simulink model "Cooperative_XeYe"  (Simulink 9.1)
settings: Solver=ode45  StartTime=0.0  StopTime=800  FixedStep=0.2  RelTol=1e-3
values from neighbouring files (symbols this model uses):
  A1 = 0.08    [Parameters.m]
  a1 = 10    [Parameters.m]
  A2 = 0.08    [Parameters.m]
  a2 = 10    [Parameters.m]
  A3 = 0.08    [Parameters.m]
  a3 = 10    [Parameters.m]
  H_A = 2.0    (= 2)    [Parameters.m]
  H_B = 2.0    (= 2)    [Parameters.m]
  k1_A = 5    [Parameters.m]
  k1_B = 0.1    [Parameters.m]
  k1_C = 5    [Parameters.m]
  k_update_A = 5.0    (= 5)    [Parameters.m]
  k_update_B = 10.0    (= 10)    [Parameters.m]
  k_update_C = 5.0    (= 5)    [Parameters.m]
  T = 0.2    [Parameters.m]
  v_0 = 1.0    (= 1)    [Parameters.m]
settings Model: Creator=sunky  LastModifiedBy=xiaobo
settings DataIOCC: SaveFormat=Dataset
settings OptimizationCC: LifeSpan=auto
settings DebuggingCC: UnderspecifiedInitializationDetection=Simplified  MergeDetectMultiDrivingBlocksExec=error  SFUnexpectedBacktrackingDiag=error  SFNoUnconditionalDefaultTransitionDiag=error  SFExecutionAtInitializationDiag=warning
settings HardwareCC: ProdBitPerPointer=64  ProdBitPerSizeT=64  ProdBitPerPtrDiffT=64  ProdLargestAtomicFloat=Float  ProdIntDivRoundTo=Zero  ProdEndianess=LittleEndian  ProdWordSize=64  ProdHWDeviceType=Intel->x86-64 (Windows64)
settings ModelReferenceCC: PropagateSignalLabelsOutOfModel=on
settings GRTTargetCC: TargetLangStandard=C99 (ISO)  CombineOutputUpdateFcns=on  GRTInterface=off
settings ConfigComp: CovMetricSettings=dwe  CovHtmlReporting=off  CovSaveCumulativeToWorkspaceVar=off  CovSaveSingleToWorkspaceVar=off  CovExternalEMLEnable=on

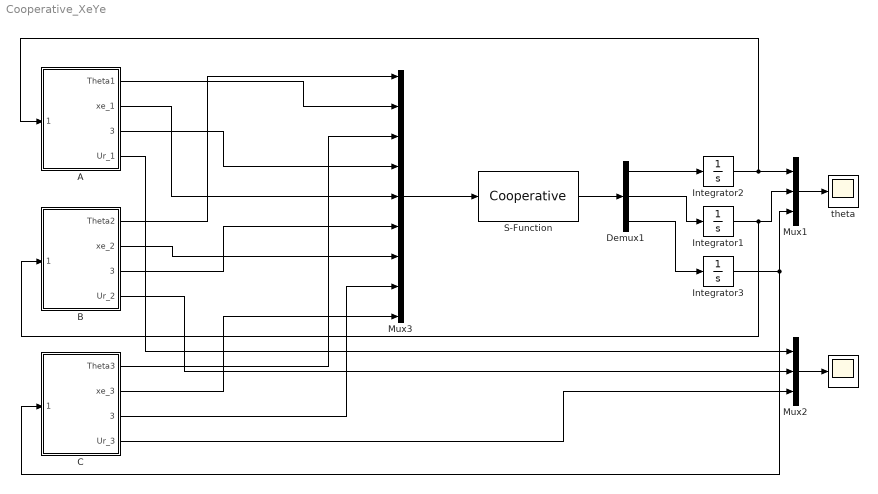
== system Cooperative_XeYe ==
  "   " : Scope
  " theta " : Scope
  A : Subsystem
  B : Subsystem
  C : Subsystem
  Demux1 : Demux  Outputs=3
  Integrator1 : Integrator
  Integrator2 : Integrator
  Integrator3 : Integrator
  Mux1 : Mux  Inputs=3
  Mux2 : Mux  Inputs=3
  Mux3 : Mux  Inputs=9
  S-Function : S-Function  FunctionName=Cooperative  Parameters=A1,A2,A3,v_0,T,a1,a2,a3  SFunctionDeploymentMode=off  EnableBusSupport=off
  wires:
  A/2(xe_1) -> Mux3/5
  A/3(u_dxing_A) -> Mux3/4
  B/2(xe_2) -> Mux3/7
  B/3(u_dxing_B) -> Mux3/6
  C/2(xe_3) -> Mux3/9
  C/3(u_dxing_C) -> Mux3/8
  Mux3/1 -> S-Function/1
  S-Function/1 -> Demux1/1
  Demux1/1 -> Integrator2/1
  Demux1/2 -> Integrator1/1
  Demux1/3 -> Integrator3/1
  Integrator2/1 -> A/1(Update1), Mux1/1
  Integrator1/1 -> B/1(Update2), Mux1/2
  Integrator3/1 -> C/1(Update3), Mux1/3
  Mux1/1 -> " theta "/1
  A/4(Ur_1) -> Mux2/1
  B/4(Ur_2) -> Mux2/2
  C/4(Ur_3) -> Mux2/3
  Mux2/1 -> "   "/1
  A/1(Theta1) -> Mux3/2
  B/1(Theta2) -> Mux3/1
  C/1(Theta3) -> Mux3/3

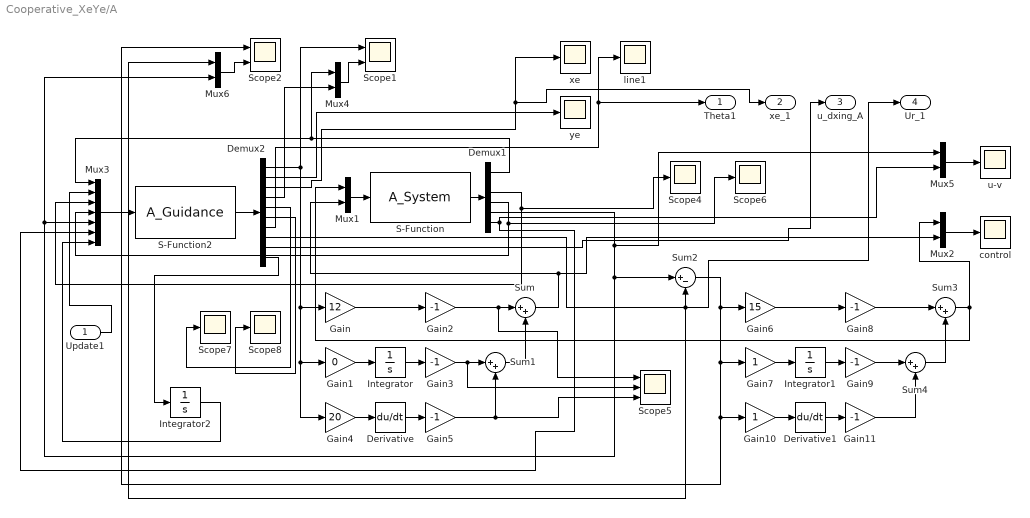
== system Cooperative_XeYe/A ==
  Update1 : Inport
  Demux1 : Demux  Outputs=6
  Demux2 : Demux  Outputs=10
  Derivative : Derivative
  Derivative1 : Derivative
  Gain : Gain  Gain=12
  Gain1 : Gain  Gain=0
  Gain10 : Gain
  Gain{2..3,5,8..9,11} (6 alike) : Gain  Gain=-1
  Gain4 : Gain  Gain=20
  Gain6 : Gain  Gain=15
  Gain7 : Gain
  Integrator : Integrator
  Integrator1 : Integrator
  Integrator2 : Integrator
  Mux{1..2,4..6} (5 alike) : Mux  Inputs=2
  Mux3 : Mux  Inputs=7
  S-Function : S-Function  FunctionName=A_System  SFunctionDeploymentMode=off  EnableBusSupport=off
  S-Function2 : S-Function  FunctionName=A_Guidance  Parameters=H_A,v_0,k_update_A,k1_A  SFunctionDeploymentMode=off  EnableBusSupport=off
  Scope1 : Scope  NumInputPorts=2
  Scope2 : Scope  NumInputPorts=2
  Scope{4,6..8} (4 alike) : Scope
  Scope5 : Scope  NumInputPorts=3
  Sum{,1,3..4} (4 alike) : Sum  Inputs=|++
  Sum2 : Sum  Inputs=|+-
  control : Scope
  line1 : Scope
  u-v : Scope
  xe : Scope
  ye : Scope
  Theta1 : Outport
  xe_1 : Outport  Port=2
  u_dxing_A : Outport  Port=3
  Ur_1 : Outport  Port=4
  wires:
  Demux1/1 -> Mux4/1, Mux3/1
  Gain8/1 -> Sum3/1
  Derivative1/1 -> Gain11/1
  Mux3/1 -> S-Function2/1
  S-Function/1 -> Demux1/1
  Demux2/5 -> Scope7/1
  Integrator1/1 -> Gain9/1
  Gain6/1 -> Gain8/1
  Gain5/1 -> Sum1/2, Scope5/3
  Sum/1 -> Mux2/2, Mux1/2
  Mux2/1 -> control/1
  Gain3/1 -> Scope5/2, Sum1/1
  Gain2/1 -> Scope5/1, Sum/1
  Demux2/6 -> Scope8/1
  Sum2/1 -> Scope2/1, Gain10/1, Gain7/1, Gain6/1
  Gain7/1 -> Integrator1/1
  Demux2/8 -> Ur_1/1, Mux6/1, Sum2/2
  Demux1/5 -> Mux5/1, Sum2/1, Mux6/2, Mux3/5
  Sum3/1 -> Mux1/1, Mux2/1
  Gain9/1 -> Sum4/1
  Mux1/1 -> S-Function/1
  Demux2/7 -> Theta1/1, line1/1
  Gain10/1 -> Derivative1/1
  Demux1/4 -> Scope6/1, Mux3/4
  S-Function2/1 -> Demux2/1
  Integrator/1 -> Gain3/1
  Demux1/6 -> Mux3/6, Mux5/2
  Gain/1 -> Gain2/1
  Gain11/1 -> Sum4/2
  Demux2/3 -> xe_1/1, xe/1
  Mux5/1 -> u-v/1
  Demux2/9 -> u_dxing_A/1
  Mux4/1 -> Scope1/2
  Gain4/1 -> Derivative/1
  Derivative/1 -> Gain5/1
  Gain1/1 -> Integrator/1
  Mux6/1 -> Scope2/2
  Demux2/4 -> Mux4/2
  Demux2/1 -> Scope1/1, Gain4/1, Gain1/1, Gain/1
  Sum1/1 -> Sum/2
  Demux2/2 -> ye/1
  Demux1/3 -> Scope4/1, Mux3/3
  Sum4/1 -> Sum3/2
  Demux2/10 -> Integrator2/1
  Integrator2/1 -> Mux3/7
  Update1/1 -> Mux3/2

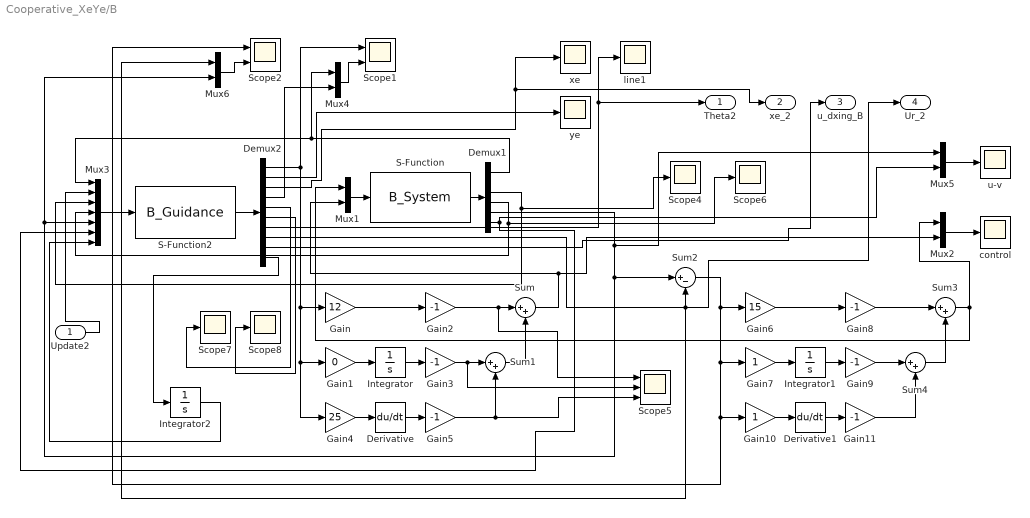
== system Cooperative_XeYe/B ==
  Update2 : Inport
  Demux1 : Demux  Outputs=6
  Demux2 : Demux  Outputs=10
  Derivative : Derivative
  Derivative1 : Derivative
  Gain : Gain  Gain=12
  Gain1 : Gain  Gain=0
  Gain10 : Gain
  Gain{2..3,5,8..9,11} (6 alike) : Gain  Gain=-1
  Gain4 : Gain  Gain=25
  Gain6 : Gain  Gain=15
  Gain7 : Gain
  Integrator : Integrator
  Integrator1 : Integrator
  Integrator2 : Integrator
  Mux{1..2,4..6} (5 alike) : Mux  Inputs=2
  Mux3 : Mux  Inputs=7
  S-Function : S-Function  FunctionName=B_System  SFunctionDeploymentMode=off  EnableBusSupport=off
  S-Function2 : S-Function  FunctionName=B_Guidance  Parameters=H_B,v_0,k_update_B,k1_B  SFunctionDeploymentMode=off  EnableBusSupport=off
  Scope1 : Scope  NumInputPorts=2
  Scope2 : Scope  NumInputPorts=2
  Scope{4,6..8} (4 alike) : Scope
  Scope5 : Scope  NumInputPorts=3
  Sum{,1,3..4} (4 alike) : Sum  Inputs=|++
  Sum2 : Sum  Inputs=|+-
  control : Scope
  line1 : Scope
  u-v : Scope
  xe : Scope
  ye : Scope
  Theta2 : Outport
  xe_2 : Outport  Port=2
  u_dxing_B : Outport  Port=3
  Ur_2 : Outport  Port=4
  wires:
  Demux1/1 -> Mux4/1, Mux3/1
  Gain8/1 -> Sum3/1
  Derivative1/1 -> Gain11/1
  Mux3/1 -> S-Function2/1
  S-Function/1 -> Demux1/1
  Demux2/5 -> Scope7/1
  Integrator1/1 -> Gain9/1
  Gain6/1 -> Gain8/1
  Gain5/1 -> Sum1/2, Scope5/3
  Sum/1 -> Mux2/2, Mux1/2
  Mux2/1 -> control/1
  Gain3/1 -> Scope5/2, Sum1/1
  Gain2/1 -> Scope5/1, Sum/1
  Demux2/6 -> Scope8/1
  Sum2/1 -> Scope2/1, Gain10/1, Gain7/1, Gain6/1
  Gain7/1 -> Integrator1/1
  Demux2/8 -> Ur_2/1, Mux6/1, Sum2/2
  Demux1/5 -> Mux5/1, Sum2/1, Mux6/2, Mux3/5
  Sum3/1 -> Mux1/1, Mux2/1
  Gain9/1 -> Sum4/1
  Mux1/1 -> S-Function/1
  Demux2/7 -> Theta2/1, line1/1
  Gain10/1 -> Derivative1/1
  Demux1/4 -> Scope6/1, Mux3/4
  S-Function2/1 -> Demux2/1
  Integrator/1 -> Gain3/1
  Demux1/6 -> Mux3/6, Mux5/2
  Gain/1 -> Gain2/1
  Gain11/1 -> Sum4/2
  Demux2/3 -> xe/1, xe_2/1
  Mux5/1 -> u-v/1
  Demux2/9 -> u_dxing_B/1
  Mux4/1 -> Scope1/2
  Gain4/1 -> Derivative/1
  Derivative/1 -> Gain5/1
  Gain1/1 -> Integrator/1
  Mux6/1 -> Scope2/2
  Demux2/4 -> Mux4/2
  Demux2/1 -> Scope1/1, Gain4/1, Gain1/1, Gain/1
  Sum1/1 -> Sum/2
  Demux2/2 -> ye/1
  Demux1/3 -> Scope4/1, Mux3/3
  Sum4/1 -> Sum3/2
  Update2/1 -> Mux3/2
  Demux2/10 -> Integrator2/1
  Integrator2/1 -> Mux3/7

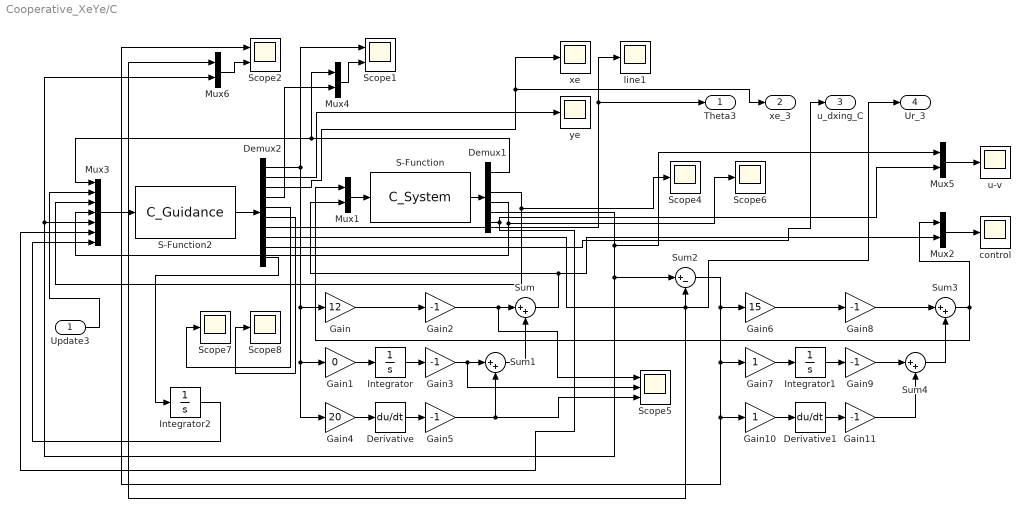
== system Cooperative_XeYe/C ==
  Update3 : Inport
  Demux1 : Demux  Outputs=6
  Demux2 : Demux  Outputs=10
  Derivative : Derivative
  Derivative1 : Derivative
  Gain : Gain  Gain=12
  Gain1 : Gain  Gain=0
  Gain10 : Gain
  Gain{2..3,5,8..9,11} (6 alike) : Gain  Gain=-1
  Gain4 : Gain  Gain=20
  Gain6 : Gain  Gain=15
  Gain7 : Gain
  Integrator : Integrator
  Integrator1 : Integrator
  Integrator2 : Integrator
  Mux{1..2,4..6} (5 alike) : Mux  Inputs=2
  Mux3 : Mux  Inputs=7
  S-Function : S-Function  FunctionName=C_System  SFunctionDeploymentMode=off  EnableBusSupport=off
  S-Function2 : S-Function  FunctionName=C_Guidance  Parameters=H_B,v_0,k_update_C,k1_C  SFunctionDeploymentMode=off  EnableBusSupport=off
  Scope1 : Scope  NumInputPorts=2
  Scope2 : Scope  NumInputPorts=2
  Scope{4,6..8} (4 alike) : Scope
  Scope5 : Scope  NumInputPorts=3
  Sum{,1,3..4} (4 alike) : Sum  Inputs=|++
  Sum2 : Sum  Inputs=|+-
  control : Scope
  line1 : Scope
  u-v : Scope
  xe : Scope
  ye : Scope
  Theta3 : Outport
  xe_3 : Outport  Port=2
  u_dxing_C : Outport  Port=3
  Ur_3 : Outport  Port=4
  wires:
  Demux1/1 -> Mux4/1, Mux3/1
  Gain8/1 -> Sum3/1
  Derivative1/1 -> Gain11/1
  Mux3/1 -> S-Function2/1
  S-Function/1 -> Demux1/1
  Demux2/5 -> Scope7/1
  Integrator1/1 -> Gain9/1
  Gain6/1 -> Gain8/1
  Gain5/1 -> Sum1/2, Scope5/3
  Sum/1 -> Mux2/2, Mux1/2
  Mux2/1 -> control/1
  Gain3/1 -> Scope5/2, Sum1/1
  Gain2/1 -> Scope5/1, Sum/1
  Demux2/6 -> Scope8/1
  Sum2/1 -> Scope2/1, Gain10/1, Gain7/1, Gain6/1
  Gain7/1 -> Integrator1/1
  Demux2/8 -> Ur_3/1, Mux6/1, Sum2/2
  Demux1/5 -> Mux5/1, Sum2/1, Mux6/2, Mux3/5
  Sum3/1 -> Mux1/1, Mux2/1
  Gain9/1 -> Sum4/1
  Mux1/1 -> S-Function/1
  Demux2/7 -> Theta3/1, line1/1
  Gain10/1 -> Derivative1/1
  Demux1/4 -> Scope6/1, Mux3/4
  S-Function2/1 -> Demux2/1
  Integrator/1 -> Gain3/1
  Demux1/6 -> Mux3/6, Mux5/2
  Gain/1 -> Gain2/1
  Gain11/1 -> Sum4/2
  Demux2/3 -> xe_3/1, xe/1
  Mux5/1 -> u-v/1
  Demux2/9 -> u_dxing_C/1
  Mux4/1 -> Scope1/2
  Gain4/1 -> Derivative/1
  Derivative/1 -> Gain5/1
  Gain1/1 -> Integrator/1
  Mux6/1 -> Scope2/2
  Demux2/4 -> Mux4/2
  Demux2/1 -> Scope1/1, Gain4/1, Gain1/1, Gain/1
  Sum1/1 -> Sum/2
  Demux2/2 -> ye/1
  Demux1/3 -> Scope4/1, Mux3/3
  Sum4/1 -> Sum3/2
  Update3/1 -> Mux3/2
  Demux2/10 -> Integrator2/1
  Integrator2/1 -> Mux3/7
